simulink library "TBCI_lib"  (Simulink 7.5)
settings: Solver=ode45  StartTime=0.0  StopTime=10.0  RelTol=1e-3
values from neighbouring files (symbols this model uses):
  pTBCI_bool_ChrgTempEnbl_C = Simulink.Parameter    [TBCI_par.m]
  pTBCI_bool_PEEnbl_C = Simulink.Parameter    [TBCI_par.m]
  pTBCI_degC_ACChrgrPlgTempHi_C = Simulink.Parameter    [TBCI_par.m]
  pTBCI_degC_DCChrgrPlgTempHi_C = Simulink.Parameter    [TBCI_par.m]
  pTBCI_mV_ChrgrUplgLwrThd_C = Simulink.Parameter    [TBCI_par.m]
  pTBCI_mV_ChrgrUplgUpprThd_C = Simulink.Parameter    [TBCI_par.m]
  pTBCI_ratio_mVtoV_C = Simulink.Parameter    [TBCI_par.m]
  pTBCI_s_ChrgPsdTiVld_C = Simulink.Parameter    [TBCI_par.m]
  pTBCI_s_TiDlyChrgrErr_C = Simulink.Parameter    [TBCI_par.m]
  pTBCI_st_ChrgConMap_C = Simulink.Parameter    [TBCI_par.m]
  pTBCI_st_ChrgDspConMap_C = Simulink.Parameter    [TBCI_par.m]
  pTBCI_V_ChrgConMapRng_C = Simulink.Parameter    [TBCI_par.m]
  pTBCI_V_ChrgDspConMapRng_C = Simulink.Parameter    [TBCI_par.m]
undefined symbols (not defined in the file or in its folder): ChrgActStsTyp, ChrgConTyp, DiscIntNeverNeededParam, p_bool_dSPaceEnbl_C, p_bool_False_M, p_bool_True_M
libraries: BaseOperationLib_Browser x51, PES_CZ_FAW x5, simulink x1
settings Model: Creator=wuaibin  LastModifiedBy=wuaibin

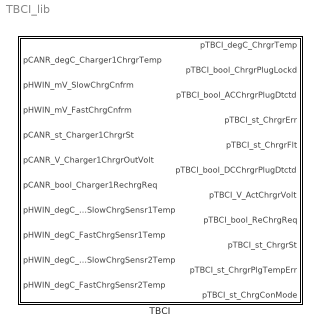
== system TBCI_lib ==
  TBCI : Subsystem  TreatAsAtomicUnit=on

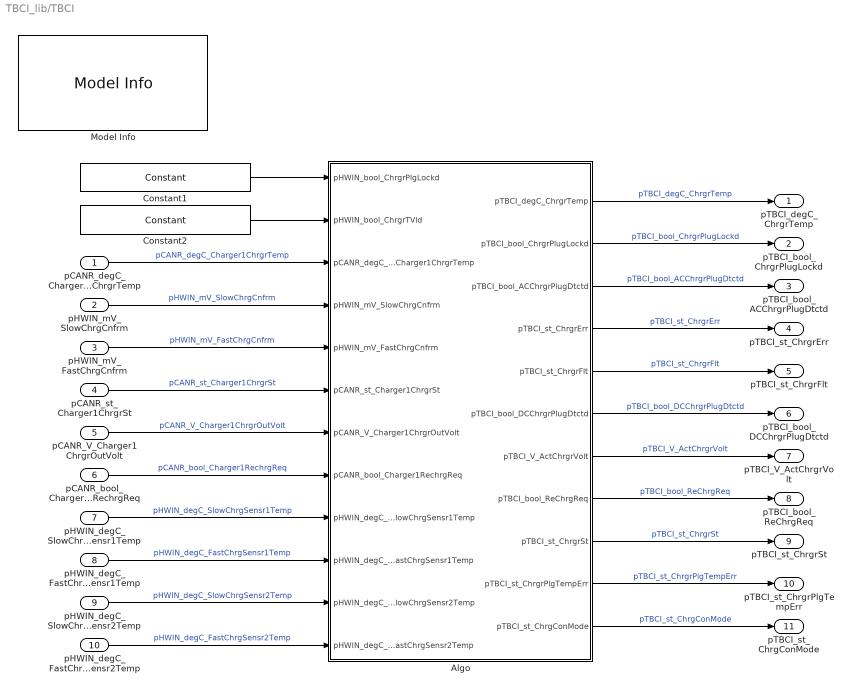
== system TBCI_lib/TBCI ==
  pCANR_degC_Charger1ChrgrTemp : Inport  OutDataType=fixdt(1, 16)  OutScaling=2^0
  pHWIN_mV_SlowChrgCnfrm : Inport  Port=2  OutDataType=fixdt(1, 16)  OutScaling=2^0
  pHWIN_mV_FastChrgCnfrm : Inport  Port=3  OutDataType=fixdt(1, 16)  OutScaling=2^0
  pCANR_st_Charger1ChrgrSt : Inport  Port=4  OutDataType=fixdt(1, 16)  OutScaling=2^0
  pCANR_V_Charger1ChrgrOutVolt : Inport  Port=5  OutDataType=fixdt(1, 16)  OutScaling=2^0
  pCANR_bool_Charger1RechrgReq : Inport  Port=6  OutDataType=fixdt(1, 16)  OutScaling=2^0
  pHWIN_degC_SlowChrgSensr1Temp : Inport  Port=7  OutDataType=fixdt(1, 16)  OutScaling=2^0
  pHWIN_degC_FastChrgSensr1Temp : Inport  Port=8  OutDataType=fixdt(1, 16)  OutScaling=2^0
  pHWIN_degC_SlowChrgSensr2Temp : Inport  Port=9  OutDataType=fixdt(1, 16)  OutScaling=2^0
  pHWIN_degC_FastChrgSensr2Temp : Inport  Port=10  OutDataType=fixdt(1, 16)  OutScaling=2^0
  Algo : Subsystem
  Constant1 : BaseOperationLib_Browser/Sources&Sinks/Constant  Value=p_bool_True_M  OutMin=[]  OutMax=[]  OutDataType=fixdt(1, 16)  ConRadixGroup=Use specified scaling  OutScaling=2^0  OutDataTypeStr=Inherit: Inherit from 'Constant value'
  Constant2 : BaseOperationLib_Browser/Sources&Sinks/Constant  Value=p_bool_True_M  OutMin=[]  OutMax=[]  OutDataType=fixdt(1, 16)  ConRadixGroup=Use specified scaling  OutScaling=2^0  OutDataTypeStr=Inherit: Inherit from 'Constant value'
  Model Info : simulink/Model-Wide Utilities/Model Info  SystemSampleTime=-1  InitialBlockCM=None  BlockCM=None  Frame=off  DisplayStringWithTags=Model Info\nCreated: %<Created>\nCreator: wuaibin  HorizontalTextAlignment=Center  LeftAlignmentValue=0.5  SourceBlockDiagram=HQEV_HCU  TagMaxNumber=20
  pTBCI_degC_ChrgrTemp : Outport  OutDataType=fixdt(1, 16)  OutScaling=2^0
  pTBCI_bool_ChrgrPlugLockd : Outport  Port=2  OutDataType=fixdt(1, 16)  OutScaling=2^0
  pTBCI_bool_ACChrgrPlugDtctd : Outport  Port=3  OutDataType=fixdt(1, 16)  OutScaling=2^0
  pTBCI_st_ChrgrErr : Outport  Port=4  OutDataType=fixdt(1, 16)  OutScaling=2^0
  pTBCI_st_ChrgrFlt : Outport  Port=5  OutDataType=fixdt(1, 16)  OutScaling=2^0
  pTBCI_bool_DCChrgrPlugDtctd : Outport  Port=6  PortDimensions=1  DataType=boolean  OutDataType=fixdt(1, 16)  OutScaling=2^0  OutDataTypeStr=boolean
  pTBCI_V_ActChrgrVolt : Outport  Port=7  OutDataType=fixdt(1, 16)  OutScaling=2^0
  pTBCI_bool_ReChrgReq : Outport  Port=8  OutDataType=fixdt(1, 16)  OutScaling=2^0
  pTBCI_st_ChrgrSt : Outport  Port=9  OutDataType=fixdt(1, 16)  OutScaling=2^0
  pTBCI_st_ChrgrPlgTempErr : Outport  Port=10  OutDataType=fixdt(1, 16)  OutScaling=2^0
  pTBCI_st_ChrgConMode : Outport  Port=11
  wires:
  Algo/11(pTBCI_st_ChrgConMode) -> pTBCI_st_ChrgConMode/1  "pTBCI_st_ChrgConMode"
  Constant2/1 -> Algo/2(pHWIN_bool_ChrgrTVld)
  Constant1/1 -> Algo/1(pHWIN_bool_ChrgrPlgLockd)
  Algo/10(pTBCI_st_ChrgrPlgTempErr) -> pTBCI_st_ChrgrPlgTempErr/1  "pTBCI_st_ChrgrPlgTempErr"
  pHWIN_degC_FastChrgSensr2Temp/1 -> Algo/12(pHWIN_degC_FastChrgSensr2Temp)  "pHWIN_degC_FastChrgSensr2Temp"
  pHWIN_degC_SlowChrgSensr2Temp/1 -> Algo/11(pHWIN_degC_SlowChrgSensr2Temp)  "pHWIN_degC_SlowChrgSensr2Temp"
  pHWIN_degC_FastChrgSensr1Temp/1 -> Algo/10(pHWIN_degC_FastChrgSensr1Temp)  "pHWIN_degC_FastChrgSensr1Temp"
  pHWIN_degC_SlowChrgSensr1Temp/1 -> Algo/9(pHWIN_degC_SlowChrgSensr1Temp)  "pHWIN_degC_SlowChrgSensr1Temp"
  pHWIN_mV_FastChrgCnfrm/1 -> Algo/5(pHWIN_mV_FastChrgCnfrm)  "pHWIN_mV_FastChrgCnfrm"
  Algo/9(pTBCI_st_ChrgrSt) -> pTBCI_st_ChrgrSt/1  "pTBCI_st_ChrgrSt"
  Algo/8(pTBCI_bool_ReChrgReq) -> pTBCI_bool_ReChrgReq/1  "pTBCI_bool_ReChrgReq"
  pCANR_bool_Charger1RechrgReq/1 -> Algo/8(pCANR_bool_Charger1RechrgReq)  "pCANR_bool_Charger1RechrgReq"
  Algo/7(pTBCI_V_ActChrgrVolt) -> pTBCI_V_ActChrgrVolt/1  "pTBCI_V_ActChrgrVolt"
  pCANR_V_Charger1ChrgrOutVolt/1 -> Algo/7(pCANR_V_Charger1ChrgrOutVolt)  "pCANR_V_Charger1ChrgrOutVolt"
  Algo/6(pTBCI_bool_DCChrgrPlugDtctd) -> pTBCI_bool_DCChrgrPlugDtctd/1  "pTBCI_bool_DCChrgrPlugDtctd"
  pCANR_degC_Charger1ChrgrTemp/1 -> Algo/3(pCANR_degC_Charger1ChrgrTemp)  "pCANR_degC_Charger1ChrgrTemp"
  pHWIN_mV_SlowChrgCnfrm/1 -> Algo/4(pHWIN_mV_SlowChrgCnfrm)  "pHWIN_mV_SlowChrgCnfrm"
  pCANR_st_Charger1ChrgrSt/1 -> Algo/6(pCANR_st_Charger1ChrgrSt)  "pCANR_st_Charger1ChrgrSt"
  Algo/1(pTBCI_degC_ChrgrTemp) -> pTBCI_degC_ChrgrTemp/1  "pTBCI_degC_ChrgrTemp"
  Algo/2(pTBCI_bool_ChrgrPlugLockd) -> pTBCI_bool_ChrgrPlugLockd/1  "pTBCI_bool_ChrgrPlugLockd"
  Algo/3(pTBCI_bool_ACChrgrPlugDtctd) -> pTBCI_bool_ACChrgrPlugDtctd/1  "pTBCI_bool_ACChrgrPlugDtctd"
  Algo/4(pTBCI_st_ChrgrErr) -> pTBCI_st_ChrgrErr/1  "pTBCI_st_ChrgrErr"
  Algo/5(pTBCI_st_ChrgrFlt) -> pTBCI_st_ChrgrFlt/1  "pTBCI_st_ChrgrFlt"

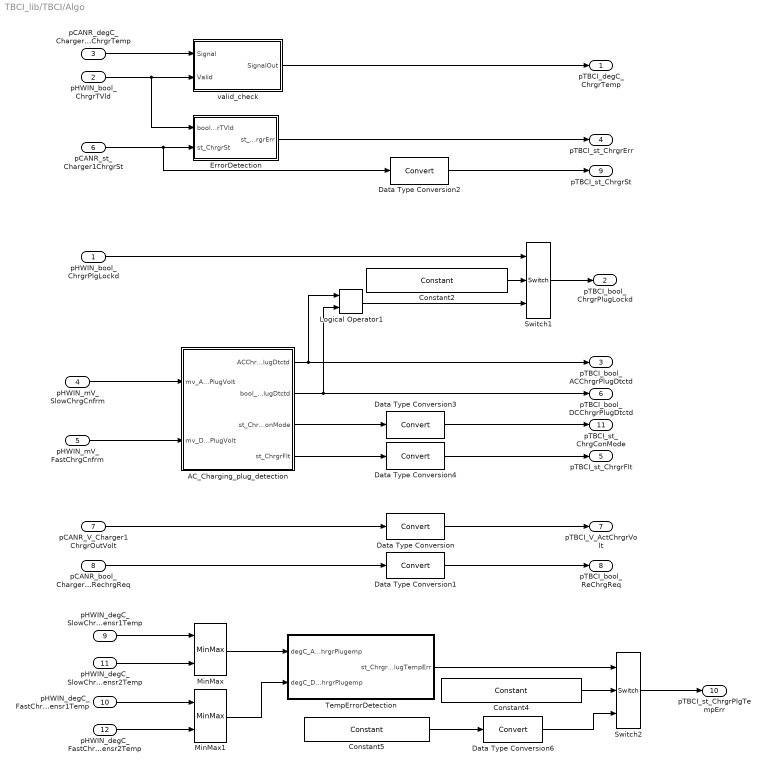
== system TBCI_lib/TBCI/Algo ==
  pHWIN_bool_ChrgrPlgLockd : Inport  OutDataType=fixdt(1, 16)  OutScaling=2^0
  pHWIN_bool_ChrgrTVld : Inport  Port=2  OutDataType=fixdt(1, 16)  OutScaling=2^0
  pCANR_degC_Charger1ChrgrTemp : Inport  Port=3  OutDataType=fixdt(1, 16)  OutScaling=2^0
  pHWIN_mV_SlowChrgCnfrm : Inport  Port=4  OutDataType=fixdt(1, 16)  OutScaling=2^0
  pHWIN_mV_FastChrgCnfrm : Inport  Port=5  OutDataType=fixdt(1, 16)  OutScaling=2^0
  pCANR_st_Charger1ChrgrSt : Inport  Port=6  OutDataType=fixdt(1, 16)  OutScaling=2^0
  pCANR_V_Charger1ChrgrOutVolt : Inport  Port=7  OutDataType=fixdt(1, 16)  OutScaling=2^0
  pCANR_bool_Charger1RechrgReq : Inport  Port=8  OutDataType=fixdt(1, 16)  OutScaling=2^0
  pHWIN_degC_SlowChrgSensr1Temp : Inport  Port=9  OutDataType=fixdt(1, 16)  OutScaling=2^0
  pHWIN_degC_FastChrgSensr1Temp : Inport  Port=10  OutDataType=fixdt(1, 16)  OutScaling=2^0
  pHWIN_degC_SlowChrgSensr2Temp : Inport  Port=11  OutDataType=fixdt(1, 16)  OutScaling=2^0
  pHWIN_degC_FastChrgSensr2Temp : Inport  Port=12  OutDataType=fixdt(1, 16)  OutScaling=2^0
  AC_Charging_plug_detection : Subsystem
  Constant2 : BaseOperationLib_Browser/Sources&Sinks/Constant  Value=pTBCI_bool_PEEnbl_C  OutMin=[]  OutMax=[]  OutDataType=fixdt(1, 16)  ConRadixGroup=Use specified scaling  OutScaling=2^0  OutDataTypeStr=Inherit: Inherit from 'Constant value'
  Constant4 : BaseOperationLib_Browser/Sources&Sinks/Constant  Value=pTBCI_bool_ChrgTempEnbl_C  OutMin=[]  OutMax=[]  OutDataType=fixdt(1, 16)  ConRadixGroup=Use specified scaling  OutScaling=2^0  OutDataTypeStr=Inherit: Inherit from 'Constant value'
  Constant5 : BaseOperationLib_Browser/Sources&Sinks/Constant  Value=p_bool_False_M  OutMin=[]  OutMax=[]  OutDataType=fixdt(1, 16)  ConRadixGroup=Use specified scaling  OutScaling=2^0  OutDataTypeStr=Inherit: Inherit from 'Constant value'
  Data Type Conversion{,1..4,6} (6 alike) : DataTypeConversion  OutDataType=fixdt(1, 16)  OutScaling=2^0
  ErrorDetection : Subsystem
  Logical Operator1 : BaseOperationLib_Browser/Logic Operations Changed/Logical Operator  Operator=OR  Inputs=2  AllPortsSameDT=on  OutDataTypeMode=Specify via dialog  LogicDataType=PDT_Bool  OutDataTypeStr=PDT_Bool
  MinMax : BaseOperationLib_Browser/Math Operations Changed/MinMax  Function=max  Inputs=2  InputSameDT=on  OutMin=[]  OutMax=[]  OutDataType=fixdt(1, 16)  OutScaling=2^0  SaturateOnIntegerOverflow=on
  MinMax1 : BaseOperationLib_Browser/Math Operations Changed/MinMax  Function=max  Inputs=2  InputSameDT=on  OutMin=[]  OutMax=[]  OutDataType=fixdt(1, 16)  OutScaling=2^0  SaturateOnIntegerOverflow=on
  Switch1 : BaseOperationLib_Browser/Signal Routing Changed/Switch  Criteria=u2 ~= 0  Threshold=1  InputSameDT=on  OutMin=[]  OutMax=[]  OutDataType=fixdt(1,16,0)  OutScaling=[]  SaturateOnIntegerOverflow=on
  Switch2 : BaseOperationLib_Browser/Signal Routing Changed/Switch  Criteria=u2 ~= 0  Threshold=1  InputSameDT=on  OutMin=[]  OutMax=[]  OutDataType=fixdt(1,16,0)  OutScaling=[]  SaturateOnIntegerOverflow=on
  TempErrorDetection : Subsystem
  valid_check : Subsystem  mask(Validity check      ){init=20}
      mask prompts: init "Init value"
      mask help:
      | Block checks, if the signal is valid. If not, signal is replaced by its
      | last valid value.
      mask Help:
      | Block checks, if the signal is valid. If not, signal is replaced by its
      | last valid value.
  pTBCI_degC_ChrgrTemp : Outport  OutDataType=fixdt(1, 16)  OutScaling=2^0
  pTBCI_bool_ChrgrPlugLockd : Outport  Port=2  OutDataType=fixdt(1, 16)  OutScaling=2^0
  pTBCI_bool_ACChrgrPlugDtctd : Outport  Port=3  OutDataType=fixdt(1, 16)  OutScaling=2^0
  pTBCI_st_ChrgrErr : Outport  Port=4  OutDataType=fixdt(1, 16)  OutScaling=2^0
  pTBCI_st_ChrgrFlt : Outport  Port=5  OutDataType=fixdt(1, 16)  OutScaling=2^0
  pTBCI_bool_DCChrgrPlugDtctd : Outport  Port=6  PortDimensions=1  DataType=boolean  OutDataType=fixdt(1, 16)  OutScaling=2^0  OutDataTypeStr=boolean
  pTBCI_V_ActChrgrVolt : Outport  Port=7  OutDataType=fixdt(1, 16)  OutScaling=2^0
  pTBCI_bool_ReChrgReq : Outport  Port=8  OutDataType=fixdt(1, 16)  OutScaling=2^0
  pTBCI_st_ChrgrSt : Outport  Port=9  OutDataType=fixdt(1, 16)  OutScaling=2^0
  pTBCI_st_ChrgrPlgTempErr : Outport  Port=10  OutDataType=fixdt(1, 16)  OutScaling=2^0
  pTBCI_st_ChrgConMode : Outport  Port=11
  wires:
  Data Type Conversion3/1 -> pTBCI_st_ChrgConMode/1
  Data Type Conversion6/1 -> Switch2/3
  Constant5/1 -> Data Type Conversion6/1
  Constant4/1 -> Switch2/2
  TempErrorDetection/1(st_ChrgrPlugTempErr) -> Switch2/1
  Switch2/1 -> pTBCI_st_ChrgrPlgTempErr/1
  MinMax1/1 -> TempErrorDetection/2(degC_DCChrgrPlugemp)
  MinMax/1 -> TempErrorDetection/1(degC_ACChrgrPlugemp)
  pHWIN_degC_FastChrgSensr2Temp/1 -> MinMax1/2
  pHWIN_degC_FastChrgSensr1Temp/1 -> MinMax1/1
  pHWIN_degC_SlowChrgSensr2Temp/1 -> MinMax/2
  pHWIN_degC_SlowChrgSensr1Temp/1 -> MinMax/1
  AC_Charging_plug_detection/3(st_ChrgConMode) -> Data Type Conversion3/1
  AC_Charging_plug_detection/2(bool_DCChrgrPlugDtctd) -> Logical Operator1/2, pTBCI_bool_DCChrgrPlugDtctd/1
  pHWIN_mV_FastChrgCnfrm/1 -> AC_Charging_plug_detection/2(mv_DCChrgrPlugVolt)
  Data Type Conversion2/1 -> pTBCI_st_ChrgrSt/1
  Data Type Conversion1/1 -> pTBCI_bool_ReChrgReq/1
  Data Type Conversion/1 -> pTBCI_V_ActChrgrVolt/1
  pCANR_bool_Charger1RechrgReq/1 -> Data Type Conversion1/1
  pCANR_V_Charger1ChrgrOutVolt/1 -> Data Type Conversion/1
  Logical Operator1/1 -> Switch1/3
  AC_Charging_plug_detection/1(ACChrgrPlugDtctd) -> pTBCI_bool_ACChrgrPlugDtctd/1, Logical Operator1/1
  pHWIN_mV_SlowChrgCnfrm/1 -> AC_Charging_plug_detection/1(mv_ACChrgrPlugVolt)
  pCANR_degC_Charger1ChrgrTemp/1 -> valid_check/1(Signal)
  pHWIN_bool_ChrgrTVld/1 -> valid_check/2(Valid), ErrorDetection/1(bool_ChrgrTVld)
  valid_check/1(SignalOut) -> pTBCI_degC_ChrgrTemp/1
  pCANR_st_Charger1ChrgrSt/1 -> Data Type Conversion2/1, ErrorDetection/2(st_ChrgrSt)
  ErrorDetection/1(st_ChrgrErr) -> pTBCI_st_ChrgrErr/1
  Switch1/1 -> pTBCI_bool_ChrgrPlugLockd/1
  Constant2/1 -> Switch1/2
  pHWIN_bool_ChrgrPlgLockd/1 -> Switch1/1
  AC_Charging_plug_detection/4(st_ChrgrFlt) -> Data Type Conversion4/1
  Data Type Conversion4/1 -> pTBCI_st_ChrgrFlt/1

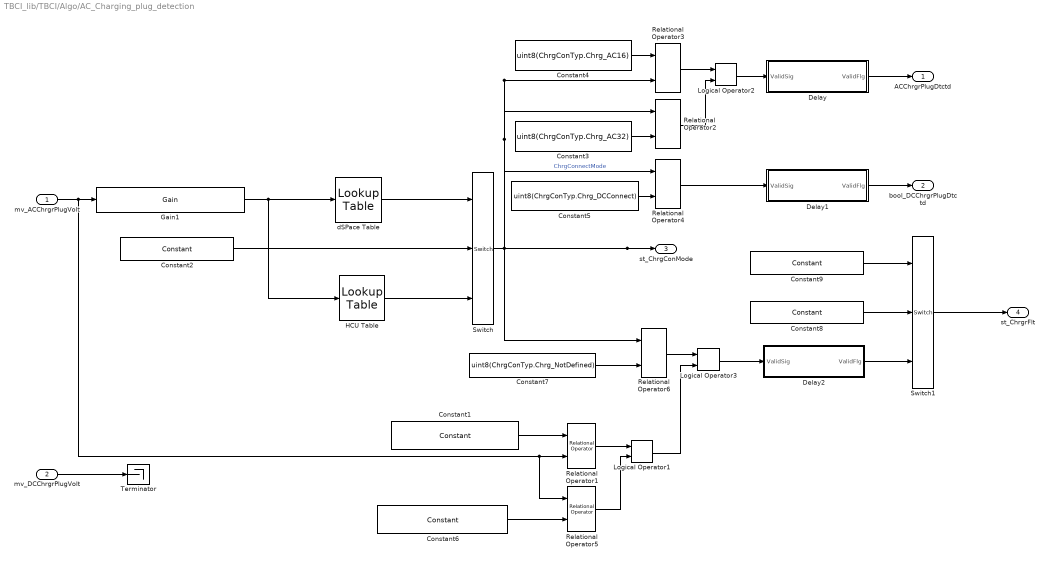
== system TBCI_lib/TBCI/Algo/AC_Charging_plug_detection ==
  mv_ACChrgrPlugVolt : Inport
  mv_DCChrgrPlugVolt : Inport  Port=2
  Constant1 : BaseOperationLib_Browser/Sources&Sinks/Constant  Value=pTBCI_mV_ChrgrUplgUpprThd_C  OutMin=[]  OutMax=[]  OutDataType=fixdt(1, 16)  ConRadixGroup=Use specified scaling  OutScaling=2^0  OutDataTypeStr=Inherit: Inherit from 'Constant value'
  Constant2 : BaseOperationLib_Browser/Sources&Sinks/Constant  Value=p_bool_dSPaceEnbl_C  OutMin=[]  OutMax=[]  OutDataType=fixdt(1, 16)  ConRadixGroup=Use specified scaling  OutScaling=2^0  OutDataTypeStr=Inherit: Inherit from 'Constant value'
  Constant3 : Constant  Value=uint8(ChrgConTyp.Chrg_AC32)  OutDataType=fixdt(1, 16)  OutScaling=2^0
      mask Display: patch([0 1 1 1 .75], [1 1 0 .75 1], [0 1 0]);
  Constant4 : Constant  Value=uint8(ChrgConTyp.Chrg_AC16)  OutDataType=fixdt(1, 16)  OutScaling=2^0
      mask Display: patch([0 1 1 1 .75], [1 1 0 .75 1], [0 1 0]);
  Constant5 : Constant  Value=uint8(ChrgConTyp.Chrg_DCConnect)  OutDataType=fixdt(1, 16)  OutScaling=2^0
      mask Display: patch([0 1 1 1 .75], [1 1 0 .75 1], [0 1 0]);
  Constant6 : BaseOperationLib_Browser/Sources&Sinks/Constant  Value=pTBCI_mV_ChrgrUplgLwrThd_C  OutMin=[]  OutMax=[]  OutDataType=fixdt(1, 16)  ConRadixGroup=Use specified scaling  OutScaling=2^0  OutDataTypeStr=Inherit: Inherit from 'Constant value'
  Constant7 : Constant  Value=uint8(ChrgConTyp.Chrg_NotDefined)  OutDataType=fixdt(1, 16)  OutScaling=2^0
      mask Display: patch([0 1 1 1 .75], [1 1 0 .75 1], [0 1 0]);
  Constant8 : BaseOperationLib_Browser/Sources&Sinks/Constant  Value=p_bool_dSPaceEnbl_C  OutMin=[]  OutMax=[]  OutDataType=fixdt(1, 16)  ConRadixGroup=Use specified scaling  OutScaling=2^0  OutDataTypeStr=Inherit: Inherit from 'Constant value'
  Constant9 : BaseOperationLib_Browser/Sources&Sinks/Constant  Value=p_bool_False_M  OutMin=[]  OutMax=[]  OutDataType=fixdt(1, 16)  ConRadixGroup=Use specified scaling  OutScaling=2^0  OutDataTypeStr=Inherit: Inherit from 'Constant value'
  Delay : Subsystem  mask{timeoutthres=pTBCI_s_ChrgPsdTiVld_C}
      mask prompts: timeoutthres "Timeout counter Treshold"
      mask help:
      | WatchDog block
      |
      | If input bool signal is false for the number of step bigger than "Timeout counter Threshold" the output WatchDog signal is set to True.
      |
      | Tip. Set the thresshold to the required time in seconds devided by algorithm sampling time.
      mask Help:
      | WatchDog block
      | 
      | If input bool signal is false for the number of step bigger than "Timeout counter Threshold" the output WatchDog signal is set to True.
      | 
      | Tip. Set the thresshold to required time in second devided by sampling time.
  Delay1 : Subsystem  mask{timeoutthres=pTBCI_s_ChrgPsdTiVld_C}
      mask prompts: timeoutthres "Timeout counter Treshold"
      mask help:
      | WatchDog block
      |
      | If input bool signal is false for the number of step bigger than "Timeout counter Threshold" the output WatchDog signal is set to True.
      |
      | Tip. Set the thresshold to the required time in seconds devided by algorithm sampling time.
      mask Help:
      | WatchDog block
      | 
      | If input bool signal is false for the number of step bigger than "Timeout counter Threshold" the output WatchDog signal is set to True.
      | 
      | Tip. Set the thresshold to required time in second devided by sampling time.
  Delay2 : Subsystem  mask{timeoutthres=pTBCI_s_TiDlyChrgrErr_C}
      mask prompts: timeoutthres "Timeout counter Treshold"
      mask help:
      | WatchDog block
      |
      | If input bool signal is false for the number of step bigger than "Timeout counter Threshold" the output WatchDog signal is set to True.
      |
      | Tip. Set the thresshold to the required time in seconds devided by algorithm sampling time.
      mask Help:
      | WatchDog block
      | 
      | If input bool signal is false for the number of step bigger than "Timeout counter Threshold" the output WatchDog signal is set to True.
      | 
      | Tip. Set the thresshold to required time in second devided by sampling time.
  Gain1 : BaseOperationLib_Browser/Math Operations Changed/Gain  Gain=pTBCI_ratio_mVtoV_C  Multiplication=Element-wise(K.*u)  ParamMin=[]  ParamMax=[]  ParameterDataType=fixdt(1, 16)  ParameterScalingMode=Best Precision: Matrix-wise  ParameterScaling=2^0  ParamDataTypeStr=Inherit: Inherit from 'Gain'  OutMin=[]  OutMax=[]  OutDataType=fixdt(1, 16)  OutScaling=2^0  SaturateOnIntegerOverflow=on
  HCU Table : BaseOperationLib_Browser/Lookup Tables Changed/Lookup Table  InputValues=pTBCI_V_ChrgConMapRng_C  Table=pTBCI_st_ChrgConMap_C  LookUpMeth=Use Input Below  OutMin=[]  OutMax=[]  OutDataTypeMode=uint8  OutDataType=fixdt(1, 16)  OutScaling=2^0  OutDataTypeStr=uint8  SaturateOnIntegerOverflow=on
      settings: AttributesFormatString=X:%<InputValues>\nTAB:%<Table>
  Logical Operator1 : BaseOperationLib_Browser/Logic Operations Changed/Logical Operator  Operator=OR  Inputs=2  AllPortsSameDT=on  OutDataTypeMode=Specify via dialog  LogicDataType=PDT_Bool  OutDataTypeStr=PDT_Bool
  Logical Operator2 : BaseOperationLib_Browser/Logic Operations Changed/Logical Operator  Operator=OR  Inputs=2  AllPortsSameDT=on  OutDataTypeMode=Specify via dialog  LogicDataType=PDT_Bool  OutDataTypeStr=PDT_Bool
  Logical Operator3 : BaseOperationLib_Browser/Logic Operations Changed/Logical Operator  Operator=OR  Inputs=2  AllPortsSameDT=on  OutDataTypeMode=Specify via dialog  LogicDataType=PDT_Bool  OutDataTypeStr=PDT_Bool
  Relational Operator1 : BaseOperationLib_Browser/Logic Operations Changed/Relational Operator  Operator=<  InputSameDT=on  LogicOutDataTypeMode=Specify via dialog  LogicDataType=PDT_Bool  OutDataTypeStr=PDT_Bool
  Relational Operator{2..4,6} (4 alike) : BaseOperationLib_Browser/Logic Operations Changed/Relational Operator  Operator===  InputSameDT=on  LogicOutDataTypeMode=Specify via dialog  LogicDataType=PDT_Bool  OutDataTypeStr=PDT_Bool
  Relational Operator5 : BaseOperationLib_Browser/Logic Operations Changed/Relational Operator  Operator=<  InputSameDT=on  LogicOutDataTypeMode=Specify via dialog  LogicDataType=PDT_Bool  OutDataTypeStr=PDT_Bool
  Switch : BaseOperationLib_Browser/Signal Routing Changed/Switch  Criteria=u2 ~= 0  Threshold=1  InputSameDT=on  OutMin=[]  OutMax=[]  OutDataType=fixdt(1,16,0)  OutScaling=[]  SaturateOnIntegerOverflow=on
  Switch1 : BaseOperationLib_Browser/Signal Routing Changed/Switch  Criteria=u2 ~= 0  Threshold=1  InputSameDT=on  OutMin=[]  OutMax=[]  OutDataType=fixdt(1,16,0)  OutScaling=[]  SaturateOnIntegerOverflow=on
  Terminator : Terminator
  dSPace Table : BaseOperationLib_Browser/Lookup Tables Changed/Lookup Table  InputValues=pTBCI_V_ChrgDspConMapRng_C  Table=pTBCI_st_ChrgDspConMap_C  LookUpMeth=Interpolation-Use End Values  OutMin=[]  OutMax=[]  OutDataTypeMode=uint8  OutDataType=fixdt(1, 16)  OutScaling=2^0  OutDataTypeStr=uint8  SaturateOnIntegerOverflow=on
      settings: AttributesFormatString=X:%<InputValues>\nTAB:%<Table>
  ACChrgrPlugDtctd : Outport
  bool_DCChrgrPlugDtctd : Outport  Port=2
  st_ChrgConMode : Outport  Port=3
  st_ChrgrFlt : Outport  Port=4
  wires:
  Constant1/1 -> Relational Operator1/1
  Constant9/1 -> Switch1/1
  Switch1/1 -> st_ChrgrFlt/1
  Constant8/1 -> Switch1/2
  Delay2/1(ValidFlg) -> Switch1/3
  Constant5/1 -> Relational Operator4/2
  Relational Operator4/1 -> Delay1/1(ValidSig)
  Relational Operator6/1 -> Logical Operator3/1
  Constant7/1 -> Relational Operator6/2
  Logical Operator3/1 -> Delay2/1(ValidSig)
  Logical Operator1/1 -> Logical Operator3/2
  Relational Operator5/1 -> Logical Operator1/2
  Relational Operator1/1 -> Logical Operator1/1
  Constant6/1 -> Relational Operator5/2
  mv_DCChrgrPlugVolt/1 -> Terminator/1
  Delay1/1(ValidFlg) -> bool_DCChrgrPlugDtctd/1
  Delay/1(ValidFlg) -> ACChrgrPlugDtctd/1
  Logical Operator2/1 -> Delay/1(ValidSig)
  Relational Operator2/1 -> Logical Operator2/2
  Relational Operator3/1 -> Logical Operator2/1
  Constant4/1 -> Relational Operator3/1
  Constant3/1 -> Relational Operator2/2
  Switch/1 -> Relational Operator6/1, Relational Operator4/1, Relational Operator3/2, Relational Operator2/1, st_ChrgConMode/1  "ChrgConnectMode"
  Constant2/1 -> Switch/2
  Gain1/1 -> HCU Table/1, dSPace Table/1
  HCU Table/1 -> Switch/3
  mv_ACChrgrPlugVolt/1 -> Relational Operator1/2, Relational Operator5/1, Gain1/1
  dSPace Table/1 -> Switch/1

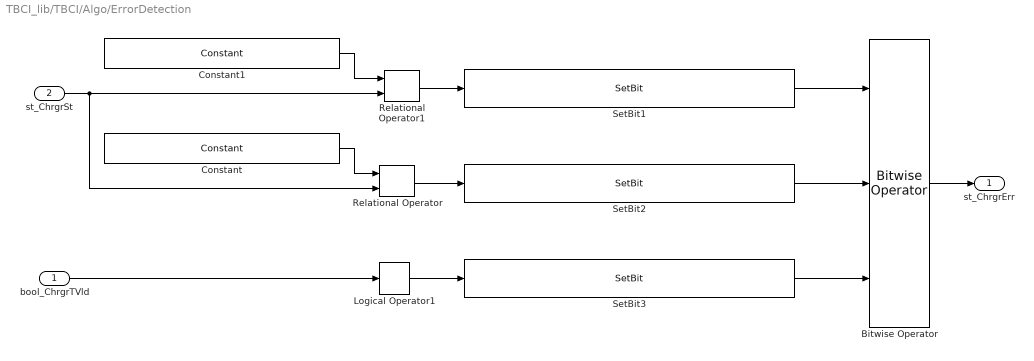
== system TBCI_lib/TBCI/Algo/ErrorDetection ==
  bool_ChrgrTVld : Inport
  st_ChrgrSt : Inport  Port=2
  Bitwise Operator : BaseOperationLib_Browser/Others Unchanged/Bitwise Operator  logicop=OR  UseBitMask=off  NumInputPorts=3  BitMask=bin2dec('11011001')  BitMaskRealWorld=Stored Integer
  Constant : BaseOperationLib_Browser/Sources&Sinks/Constant  Value=uint8(ChrgActStsTyp.ABNORMAL_FAULT)  OutMin=[]  OutMax=[]  OutDataType=fixdt(1, 16)  ConRadixGroup=Use specified scaling  OutScaling=2^0  OutDataTypeStr=Inherit: Inherit from 'Constant value'
  Constant1 : BaseOperationLib_Browser/Sources&Sinks/Constant  Value=uint8(ChrgActStsTyp.FAULT)  OutMin=[]  OutMax=[]  OutDataType=fixdt(1, 16)  ConRadixGroup=Use specified scaling  OutScaling=2^0  OutDataTypeStr=Inherit: Inherit from 'Constant value'
  Logical Operator1 : BaseOperationLib_Browser/Logic Operations Changed/Logical Operator  Operator=NOT  Inputs=2  AllPortsSameDT=on  OutDataTypeMode=Specify via dialog  LogicDataType=PDT_Bool  OutDataTypeStr=PDT_Bool
  Relational Operator : BaseOperationLib_Browser/Logic Operations Changed/Relational Operator  Operator===  InputSameDT=on  LogicOutDataTypeMode=Specify via dialog  LogicDataType=PDT_Bool  OutDataTypeStr=PDT_Bool
  Relational Operator1 : BaseOperationLib_Browser/Logic Operations Changed/Relational Operator  Operator===  InputSameDT=on  LogicOutDataTypeMode=Specify via dialog  LogicDataType=PDT_Bool  OutDataTypeStr=PDT_Bool
  SetBit1 : PES_CZ_FAW/Discontinuities/SetBit  SystemSampleTime=-1  maska=FAWChrgrErrTyp.CHARGER_ERROR
  SetBit2 : PES_CZ_FAW/Discontinuities/SetBit  SystemSampleTime=-1  maska=FAWChrgrErrTyp.CHARGER_ABNORMAL
  SetBit3 : PES_CZ_FAW/Discontinuities/SetBit  SystemSampleTime=-1  maska=FAWChrgrErrTyp.CHARGER_TEMPERATURE_INVALID
  st_ChrgrErr : Outport
  wires:
  Bitwise Operator/1 -> st_ChrgrErr/1
  Relational Operator/1 -> SetBit2/1
  Relational Operator1/1 -> SetBit1/1
  Constant1/1 -> Relational Operator1/1
  st_ChrgrSt/1 -> Relational Operator1/2, Relational Operator/2
  Constant/1 -> Relational Operator/1
  bool_ChrgrTVld/1 -> Logical Operator1/1
  SetBit1/1 -> Bitwise Operator/1
  SetBit2/1 -> Bitwise Operator/2
  SetBit3/1 -> Bitwise Operator/3
  Logical Operator1/1 -> SetBit3/1

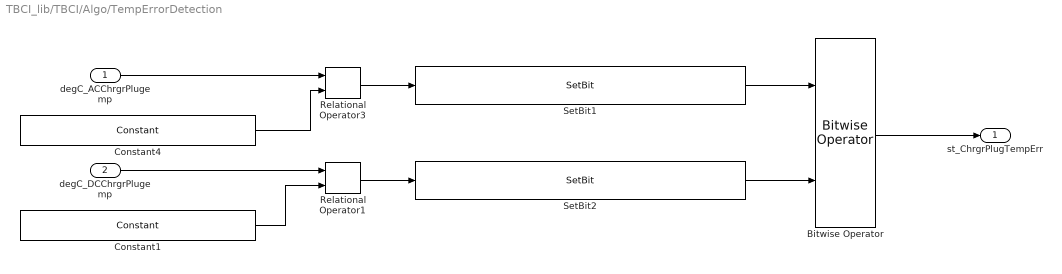
== system TBCI_lib/TBCI/Algo/TempErrorDetection ==
  degC_ACChrgrPlugemp : Inport  OutDataType=fixdt(1, 16)  OutScaling=2^0
  degC_DCChrgrPlugemp : Inport  Port=2  OutDataType=fixdt(1, 16)  OutScaling=2^0
  Bitwise Operator : BaseOperationLib_Browser/Others Unchanged/Bitwise Operator  logicop=OR  UseBitMask=off  NumInputPorts=2  BitMask=bin2dec('11011001')  BitMaskRealWorld=Stored Integer
  Constant1 : BaseOperationLib_Browser/Sources&Sinks/Constant  Value=pTBCI_degC_DCChrgrPlgTempHi_C  OutMin=[]  OutMax=[]  OutDataType=fixdt(1, 16)  ConRadixGroup=Use specified scaling  OutScaling=2^0  OutDataTypeStr=Inherit: Inherit from 'Constant value'
  Constant4 : BaseOperationLib_Browser/Sources&Sinks/Constant  Value=pTBCI_degC_ACChrgrPlgTempHi_C  OutMin=[]  OutMax=[]  OutDataType=fixdt(1, 16)  ConRadixGroup=Use specified scaling  OutScaling=2^0  OutDataTypeStr=Inherit: Inherit from 'Constant value'
  Relational Operator1 : BaseOperationLib_Browser/Logic Operations Changed/Relational Operator  Operator=>=  InputSameDT=on  LogicOutDataTypeMode=Specify via dialog  LogicDataType=PDT_Bool  OutDataTypeStr=PDT_Bool
  Relational Operator3 : BaseOperationLib_Browser/Logic Operations Changed/Relational Operator  Operator=>=  InputSameDT=on  LogicOutDataTypeMode=Specify via dialog  LogicDataType=PDT_Bool  OutDataTypeStr=PDT_Bool
  SetBit1 : PES_CZ_FAW/Discontinuities/SetBit  SystemSampleTime=-1  maska=ChrgrPlgTempHiErrTyp.CPT_ACPlgTempHi
  SetBit2 : PES_CZ_FAW/Discontinuities/SetBit  SystemSampleTime=-1  maska=ChrgrPlgTempHiErrTyp.CPT_DCPlgTempHi
  st_ChrgrPlugTempErr : Outport
  wires:
  Relational Operator1/1 -> SetBit2/1
  Relational Operator3/1 -> SetBit1/1
  Constant1/1 -> Relational Operator1/2
  degC_DCChrgrPlugemp/1 -> Relational Operator1/1
  degC_ACChrgrPlugemp/1 -> Relational Operator3/1
  SetBit2/1 -> Bitwise Operator/2
  SetBit1/1 -> Bitwise Operator/1
  Bitwise Operator/1 -> st_ChrgrPlugTempErr/1
  Constant4/1 -> Relational Operator3/2

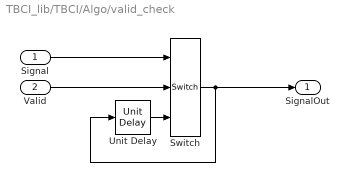
== system TBCI_lib/TBCI/Algo/valid_check ==
  Signal : Inport
  Valid : Inport  Port=2
  Switch : BaseOperationLib_Browser/Signal Routing Changed/Switch  Criteria=u2 ~= 0  Threshold=1  InputSameDT=on  OutMin=[]  OutMax=[]  OutDataType=fixdt(1,16,0)  OutScaling=[]  SaturateOnIntegerOverflow=on
  Unit Delay : BaseOperationLib_Browser/Discrete Unchanged /Unit Delay  X0=init  SampleTime=-1
  SignalOut : Outport
  wires:
  Valid/1 -> Switch/2
  Signal/1 -> Switch/1
  Unit Delay/1 -> Switch/3
  Switch/1 -> SignalOut/1, Unit Delay/1

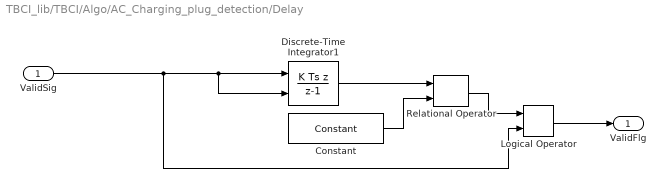
== system TBCI_lib/TBCI/Algo/AC_Charging_plug_detection/Delay ==
  ValidSig : Inport  OutDataType=fixdt(1, 16)  OutScaling=2^0
  Constant : BaseOperationLib_Browser/Sources&Sinks/Constant  Value=timeoutthres  OutMin=[]  OutMax=[]  OutDataType=fixdt(1, 16)  ConRadixGroup=Use specified scaling  OutScaling=2^0  OutDataTypeStr=Inherit: Inherit from 'Constant value'
  Discrete-Time Integrator1 : DiscreteIntegrator  IntegratorMethod=Integration: Backward Euler  ExternalReset=rising  SampleTime=-1  OutDataType=PDT_s  OutDataTypeStr=Inherit: Inherit via back propagation  UpperSaturationLimit=100  LowerSaturationLimit=0  ICPrevOutput=DiscIntNeverNeededParam  ICPrevScaledInput=DiscIntNeverNeededParam
  Logical Operator : BaseOperationLib_Browser/Logic Operations Changed/Logical Operator  Operator=AND  Inputs=2  AllPortsSameDT=on  OutDataTypeMode=Specify via dialog  LogicDataType=PDT_Bool  OutDataTypeStr=PDT_Bool
  Relational Operator : BaseOperationLib_Browser/Logic Operations Changed/Relational Operator  Operator=>=  InputSameDT=on  LogicOutDataTypeMode=Specify via dialog  LogicDataType=PDT_Bool  OutDataTypeStr=PDT_Bool
  ValidFlg : Outport  OutDataType=fixdt(1, 16)  OutScaling=2^0
  wires:
  Discrete-Time Integrator1/1 -> Relational Operator/1
  Constant/1 -> Relational Operator/2
  Logical Operator/1 -> ValidFlg/1
  Relational Operator/1 -> Logical Operator/1
  ValidSig/1 -> Logical Operator/2, Discrete-Time Integrator1/2, Discrete-Time Integrator1/1

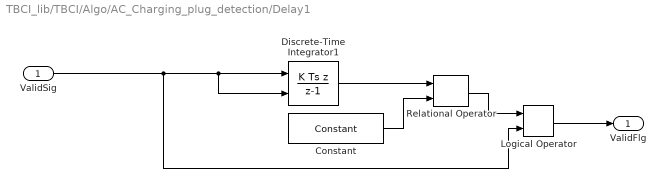
== system TBCI_lib/TBCI/Algo/AC_Charging_plug_detection/Delay1 ==
  ValidSig : Inport  OutDataType=fixdt(1, 16)  OutScaling=2^0
  Constant : BaseOperationLib_Browser/Sources&Sinks/Constant  Value=timeoutthres  OutMin=[]  OutMax=[]  OutDataType=fixdt(1, 16)  ConRadixGroup=Use specified scaling  OutScaling=2^0  OutDataTypeStr=Inherit: Inherit from 'Constant value'
  Discrete-Time Integrator1 : DiscreteIntegrator  IntegratorMethod=Integration: Backward Euler  ExternalReset=rising  SampleTime=-1  OutDataType=PDT_s  OutDataTypeStr=Inherit: Inherit via back propagation  UpperSaturationLimit=100  LowerSaturationLimit=0  ICPrevOutput=DiscIntNeverNeededParam  ICPrevScaledInput=DiscIntNeverNeededParam
  Logical Operator : BaseOperationLib_Browser/Logic Operations Changed/Logical Operator  Operator=AND  Inputs=2  AllPortsSameDT=on  OutDataTypeMode=Specify via dialog  LogicDataType=PDT_Bool  OutDataTypeStr=PDT_Bool
  Relational Operator : BaseOperationLib_Browser/Logic Operations Changed/Relational Operator  Operator=>=  InputSameDT=on  LogicOutDataTypeMode=Specify via dialog  LogicDataType=PDT_Bool  OutDataTypeStr=PDT_Bool
  ValidFlg : Outport  OutDataType=fixdt(1, 16)  OutScaling=2^0
  wires:
  ValidSig/1 -> Discrete-Time Integrator1/1, Discrete-Time Integrator1/2, Logical Operator/2
  Relational Operator/1 -> Logical Operator/1
  Logical Operator/1 -> ValidFlg/1
  Constant/1 -> Relational Operator/2
  Discrete-Time Integrator1/1 -> Relational Operator/1

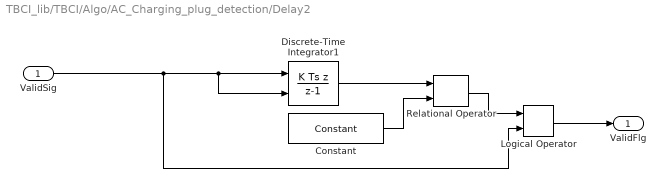
== system TBCI_lib/TBCI/Algo/AC_Charging_plug_detection/Delay2 ==
  ValidSig : Inport  OutDataType=fixdt(1, 16)  OutScaling=2^0
  Constant : BaseOperationLib_Browser/Sources&Sinks/Constant  Value=timeoutthres  OutMin=[]  OutMax=[]  OutDataType=fixdt(1, 16)  ConRadixGroup=Use specified scaling  OutScaling=2^0  OutDataTypeStr=Inherit: Inherit from 'Constant value'
  Discrete-Time Integrator1 : DiscreteIntegrator  IntegratorMethod=Integration: Backward Euler  ExternalReset=rising  SampleTime=-1  OutDataType=PDT_s  OutDataTypeStr=Inherit: Inherit via back propagation  UpperSaturationLimit=100  LowerSaturationLimit=0  ICPrevOutput=DiscIntNeverNeededParam  ICPrevScaledInput=DiscIntNeverNeededParam
  Logical Operator : BaseOperationLib_Browser/Logic Operations Changed/Logical Operator  Operator=AND  Inputs=2  AllPortsSameDT=on  OutDataTypeMode=Specify via dialog  LogicDataType=PDT_Bool  OutDataTypeStr=PDT_Bool
  Relational Operator : BaseOperationLib_Browser/Logic Operations Changed/Relational Operator  Operator=>=  InputSameDT=on  LogicOutDataTypeMode=Specify via dialog  LogicDataType=PDT_Bool  OutDataTypeStr=PDT_Bool
  ValidFlg : Outport  OutDataType=fixdt(1, 16)  OutScaling=2^0
  wires:
  Discrete-Time Integrator1/1 -> Relational Operator/1
  Constant/1 -> Relational Operator/2
  Logical Operator/1 -> ValidFlg/1
  Relational Operator/1 -> Logical Operator/1
  ValidSig/1 -> Logical Operator/2, Discrete-Time Integrator1/2, Discrete-Time Integrator1/1
